simulink model "chap8_23sim"  (Simulink 7.7)
settings: Solver=ode45  StartTime=0.0  StopTime=3  RelTol=1e-3
settings Model: Creator=ljk  LastModifiedBy=ljk

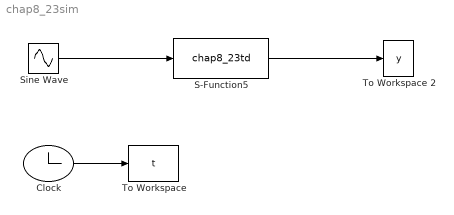
== system chap8_23sim ==
  Clock : Clock
      settings: Decimation=10
  S-Function5 : S-Function  FunctionName=chap8_23td  EnableBusSupport=off
  Sine Wave : Sin  Frequency=2*pi  SampleTime=0
  To Workspace : ToWorkspace  VariableName=t  SampleTime=-1  SaveFormat=Array
  To Workspace 2 : ToWorkspace  VariableName=y  SampleTime=-1  SaveFormat=Array
  wires:
  Sine Wave/1 -> S-Function5/1
  S-Function5/1 -> To Workspace 2/1
  Clock/1 -> To Workspace/1
